simulink model "Luenberger_Observer"  (R2022b)
settings: Solver=VariableStepAuto  StartTime=0.0  StopTime=20  RelTol=1e-3
settings Model: Creator=31904  LastModifiedBy=31904

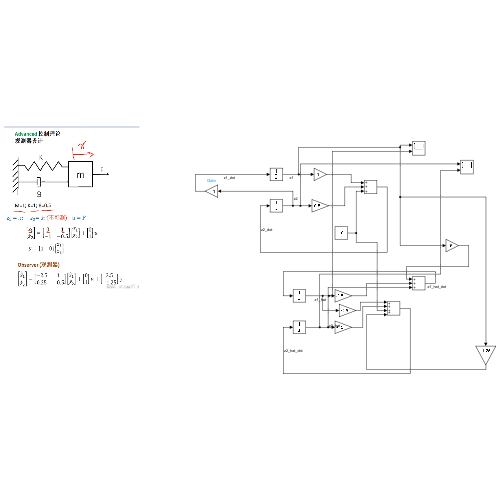
[thumbnail: Simulink's stored preview of the top-level diagram]
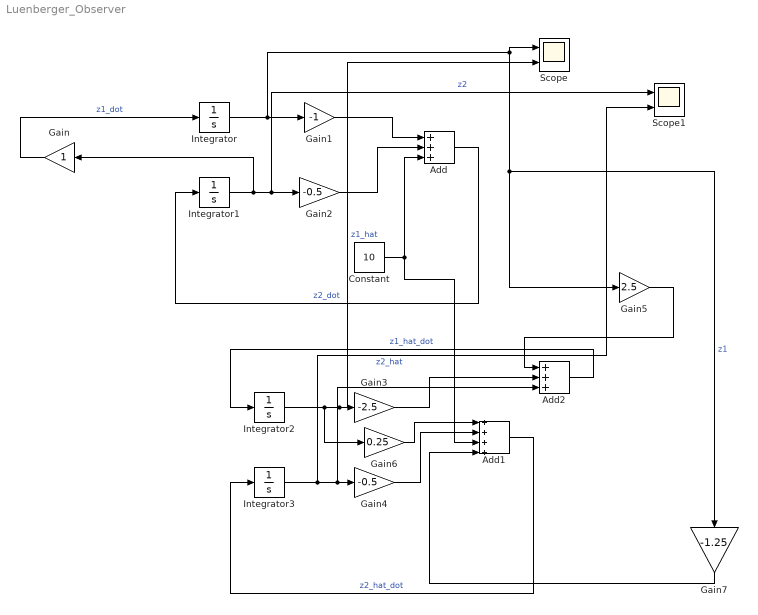
== system Luenberger_Observer ==
  Add : Sum  Inputs=+++
  Add1 : Sum  Inputs=++++
  Add2 : Sum  Inputs=+++
  Constant : Constant  Value=10
  Gain : Gain
  Gain1 : Gain  Gain=-1
  Gain2 : Gain  Gain=-0.5
  Gain3 : Gain  Gain=-2.5
  Gain4 : Gain  Gain=-0.5
  Gain5 : Gain  Gain=2.5
  Gain6 : Gain  Gain=0.25
  Gain7 : Gain  Gain=-1.25
  Integrator : Integrator
  Integrator1 : Integrator
  Integrator2 : Integrator
  Integrator3 : Integrator  InitialCondition=1
  Scope : Scope  NumInputPorts=2
  Scope1 : Scope  NumInputPorts=2
  wires:
  Gain/1 -> Integrator/1  "z1_dot"
  Integrator/1 -> Gain7/1, Gain5/1, Scope/1, Gain1/1  "z1"
  Add/1 -> Integrator1/1  "z2_dot"
  Integrator1/1 -> Scope1/1, Gain2/1, Gain/1  "z2"
  Gain1/1 -> Add/1
  Gain2/1 -> Add/2
  Add1/1 -> Integrator3/1  "z2_hat_dot"
  Integrator3/1 -> Scope1/2, Add2/3, Gain4/1  "z2_hat"
  Integrator2/1 -> Scope/2, Gain3/1, Gain6/1  "z1_hat"
  Gain4/1 -> Add1/2
  Constant/1 -> Add1/3, Add/3
  Gain3/1 -> Add2/2
  Gain5/1 -> Add2/1
  Add2/1 -> Integrator2/1  "z1_hat_dot"
  Gain6/1 -> Add1/1
  Gain7/1 -> Add1/4
